simulink model "fridge"  (Simulink 7.2)
settings: Solver=ode45  StartTime=0.0  StopTime=3600*24  RelTol=1e-3
libraries: simulink x1
settings Model: Creator=repa  LastModifiedBy=DASTUD\rvanpaassen
settings DebuggingCC: StrictBusMsg=ErrorLevel1

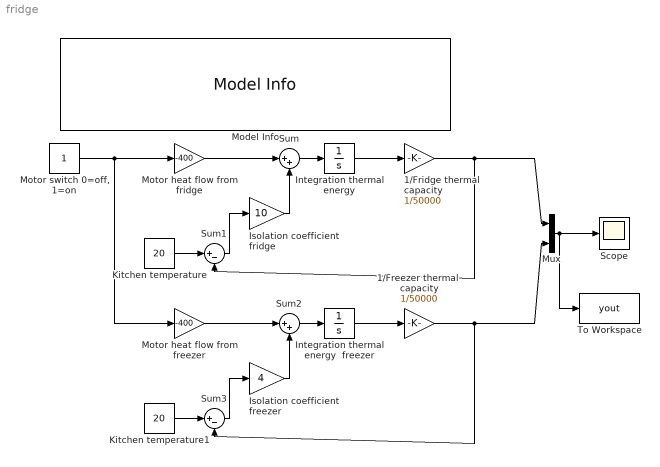
== system fridge ==
  1/Freezer thermal  capacity : Gain  Gain=1/50000
  1/Fridge thermal capacity : Gain  Gain=1/50000
  Integration thermal energy : Integrator  InitialCondition=20*50000  ContinuousStateAttributes='fridge_thermal_energy'
  Integration thermal energy  freezer : Integrator  InitialCondition=20*50000  ContinuousStateAttributes='freezer_thermal_energy'
  Isolation coefficient freezer : Gain  Gain=4
  Isolation coefficient fridge : Gain  Gain=10
  Kitchen temperature : Constant  Value=20
  Kitchen temperature1 : Constant  Value=20
  Model Info : simulink/Model-Wide Utilities/Model Info  SystemSampleTime=-1  InitialBlockCM=None  BlockCM=None  Frame=off  DisplayStringWithTags=|  HorizontalTextAlignment=Center  LeftAlignmentValue=0.5  SourceBlockDiagram=fridge  TagMaxNumber=20
      | Simple model of a refrigerator with
      | two compartments (fridge and freezer)
      | and a single motor, modeled as an idealised heat pump. 
      | Open-loop model
      | Rene van Paassen
      | version %<ModelVersion> - %<ModifiedDate>
  Motor heat flow from freezer : Gain  Gain=-400
  Motor heat flow from fridge : Gain  Gain=-400
  "Motor switch 0=off, 1=on" : Constant
  Mux : Mux  Inputs=2
  Scope : Scope
  Sum : Sum  Inputs=|++
  Sum1 : Sum  Inputs=|+-
  Sum2 : Sum  Inputs=|++
  Sum3 : Sum  Inputs=|+-
  To Workspace : ToWorkspace  VariableName=yout  SampleTime=-1  SaveFormat=Structure With Time
  wires:
  Motor heat flow from fridge/1 -> Sum/1
  "Motor switch 0=off, 1=on"/1 -> Motor heat flow from fridge/1, Motor heat flow from freezer/1
  Sum/1 -> Integration thermal energy/1
  Integration thermal energy/1 -> 1/Fridge thermal capacity/1
  Kitchen temperature/1 -> Sum1/1
  1/Fridge thermal capacity/1 -> Sum1/2, Mux/1
  Sum1/1 -> Isolation coefficient fridge/1
  Motor heat flow from freezer/1 -> Sum2/1
  Sum2/1 -> Integration thermal energy  freezer/1
  Integration thermal energy  freezer/1 -> 1/Freezer thermal  capacity/1
  Kitchen temperature1/1 -> Sum3/1
  1/Freezer thermal  capacity/1 -> Sum3/2, Mux/2
  Sum3/1 -> Isolation coefficient freezer/1
  Isolation coefficient fridge/1 -> Sum/2
  Isolation coefficient freezer/1 -> Sum2/2
  Mux/1 -> Scope/1, To Workspace/1
